simulink model "DCMotor"  (R2021a)
settings: Solver=VariableStepAuto  StartTime=0.0  StopTime=sim_time  MaxStep=step_size  RelTol=1e-3
values from neighbouring files (symbols this model uses):
  b = 3.5077E-6    (= 3.5077e-06)    [DCMotor_reduction_run.m]    (also in DCMotor_run.m; MassSpringDamper_run.m = 2; PID_ScriptOnly.m = 50; PID_SpringDamper_run.m = 10)
  J = 3.2284E-6    (= 3.2284e-06)    [DCMotor_reduction_run.m]    (also in DCMotor_run.m)
  Kb = 0.0274    [DCMotor_reduction_run.m]    (also in DCMotor_run.m)
  Kt = 0.0274    [DCMotor_reduction_run.m]    (also in DCMotor_run.m)
  L = 2.75E-6    (= 2.75e-06)    [DCMotor_reduction_run.m]    (also in DCMotor_run.m)
  R = 4    [DCMotor_reduction_run.m]    (also in DCMotor_run.m; OCV_PRC.m = 0.1)
  V = 1    [DCMotor_reduction_run.m]    (also in DCMotor_run.m; OCV_PRC.m = K0 - R * I(k) - K1/SOC - K2 * SOC + K3 * log(SOC) + K4 * log)
settings Model: Creator=shinyh  LastModifiedBy=shinyh

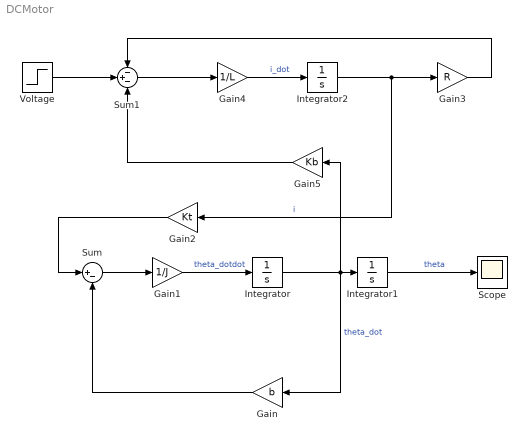
== system DCMotor ==
  Gain : Gain  Gain=b
  Gain1 : Gain  Gain=1/J
  Gain2 : Gain  Gain=Kt
  Gain3 : Gain  Gain=R
  Gain4 : Gain  Gain=1/L
  Gain5 : Gain  Gain=Kb
  Integrator : Integrator
  Integrator1 : Integrator
  Integrator2 : Integrator
  Scope : Scope
  Sum : Sum  Inputs=|+-
  Sum1 : Sum  Inputs=-+-
  Voltage : Step  After=V  SampleTime=0
  wires:
  Gain1/1 -> Integrator/1  "theta_dotdot"
  Integrator/1 -> Gain5/1, Gain/1, Integrator1/1  "theta_dot"
  Integrator1/1 -> Scope/1  "theta"
  Gain/1 -> Sum/2
  Sum/1 -> Gain1/1
  Integrator2/1 -> Gain3/1, Gain2/1  "i"
  Sum1/1 -> Gain4/1
  Gain2/1 -> Sum/1
  Gain3/1 -> Sum1/1
  Gain4/1 -> Integrator2/1  "i_dot"
  Voltage/1 -> Sum1/2
  Gain5/1 -> Sum1/3
